simulink model "Sim_Modell_hydraulisches_System_2015a"  (R2015a)
settings: Solver=ode15s  StartTime=0.0  StopTime=10  RelTol=1e-6  AbsTol=1e-5
InitFcn:
  | Parameter_hydraulisches_System
undefined symbols (not defined in the file or in its folder): parImp, parRegA, parRegoA, parSys
libraries: simulink x4, cstblocks x2
settings Model: Creator=wke  LastModifiedBy=danielhauer
settings DataIOCC: SignalLoggingSaveFormat=ModelDataLogs
settings OptimizationCC: ExpressionDepthLimit=2147483647  InitFltsAndDblsToZero=on
settings DebuggingCC: UnderspecifiedInitializationDetection=Classic  MergeDetectMultiDrivingBlocksExec=none  SolverPrmCheckMsg=warning  FcnCallInpInsideContextMsg=UseLocalSettings  StateNameClashWarn=warning
settings SFSimCC: SimParseCustomCode=off
settings GRTTargetCC: CombineOutputUpdateFcns=off  GRTInterface=on

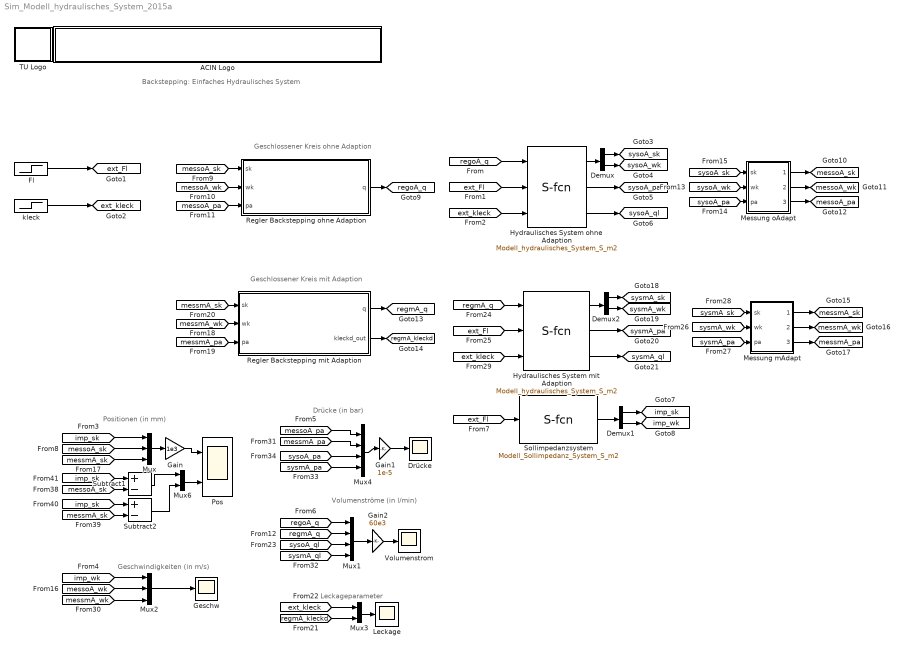
== system Sim_Modell_hydraulisches_System_2015a ==
  note: Positionen (in mm)
  note: Geschwindigkeiten (in m/s)
  note: Drücke (in bar)
  note: Leckageparameter
  note: Volumenströme (in l/min)
  note: Geschlossener Kreis ohne Adaption
  note: Geschlossener Kreis mit Adaption
  note: Backstepping: Einfaches Hydraulisches System
  ACIN Logo : Subsystem
      mask init:
      | s = get_param(gcb,'UserData');
      mask Display:
      | image(s.logo,[0 0 439 45]);
      | %axis image
  Demux : Demux  Outputs=2
  Demux1 : Demux  Outputs=2
  Demux2 : Demux  Outputs=2
  Drücke : Scope
      settings: TimeRange=auto  MaxDataPoints=5000  SaveToWorkspace=off  SaveName=ScopeData2  YMin=-10  YMax=10  SampleTime=-1
  Fl : Step  Time=3  After=1e4  SampleTime=0
  Gain : Gain  Gain=1e3
  Gain1 : Gain  Gain=1e-5
  Gain2 : Gain  Gain=60e3
  Geschw : Scope
      settings: TimeRange=auto  MaxDataPoints=5000  SaveToWorkspace=off  YMin=-10  YMax=10  SampleTime=-1
  "Hydraulisches System mit Adaption " : M-S-Function  FunctionName=Modell_hydraulisches_System_S_m2  Parameters=Aa_par,Ab_par,V0a_par,pb_par,beta_par,dk_par,m_par,sk0_par,wk0_par,pa0_par  mask{Aa_par=parSys.Aa, Ab_par=parSys.Ab, V0a_par=parSys.V0a, pb_par=parSys.pb, beta_par=parSys.beta, dk_par=parSys.dk, m_par=parSys.m, sk0_par=parSys.sk0, wk0_par=parSys.wk0, pa0_par=parSys.pa0}
      mask prompts: Aa_par "Druckwirksame Fläche Kolbenseite"; Ab_par "Druckwirksame Fläche Stangenseite"; V0a_par "eff. Volumen Kolbenseite für sk=0"; pb_par "Vorspanndruck Stangeseite"; beta_par "Kompressionsmodul"; dk_par "visk. Reibung des Kolbens"; m_par "eff. Masse des Kolbens mit Last"; sk0_par "Anfangsbedingung sk"; wk0_par "Anfangsbedingung wk"; pa0_par "Anfangsbedingung pa"
      mask Display:
      | port_label('input',1,'q');
      | port_label('input',2,'Fl');
      | port_label('input',3,'kl');
      | port_label('output',1,'sk, wk');
      | port_label('output',2,'pa');
      | port_label('output',3,'ql');
  Hydraulisches System ohne Adaption : M-S-Function  FunctionName=Modell_hydraulisches_System_S_m2  Parameters=Aa_par,Ab_par,V0a_par,pb_par,beta_par,dk_par,m_par,sk0_par,wk0_par,pa0_par  mask{Aa_par=parSys.Aa, Ab_par=parSys.Ab, V0a_par=parSys.V0a, pb_par=parSys.pb, beta_par=parSys.beta, dk_par=parSys.dk, m_par=parSys.m, sk0_par=parSys.sk0, wk0_par=parSys.wk0, pa0_par=parSys.pa0}
      mask prompts: Aa_par "Druckwirksame Fläche Kolbenseite"; Ab_par "Druckwirksame Fläche Stangenseite"; V0a_par "eff. Volumen Kolbenseite für sk=0"; pb_par "Vorspanndruck Stangeseite"; beta_par "Kompressionsmodul"; dk_par "visk. Reibung des Kolbens"; m_par "eff. Masse des Kolbens mit Last"; sk0_par "Anfangsbedingung sk"; wk0_par "Anfangsbedingung wk"; pa0_par "Anfangsbedingung pa"
      mask Display:
      | port_label('input',1,'q');
      | port_label('input',2,'Fl');
      | port_label('input',3,'kl');
      | port_label('output',1,'sk, wk');
      | port_label('output',2,'pa');
      | port_label('output',3,'ql');
  Leckage : Scope
      settings: TimeRange=auto  MaxDataPoints=5000  SaveToWorkspace=off  SaveName=ScopeData8  YMin=1.6e-012  YMax=3.9e-012  SampleTime=-1
  Messung mAdapt : Subsystem  mask{rauschenein_par=off, rauschampl_sk=5e-4, rauschampl_pa=5e4}
      mask prompts: rauschenein_par "Rauschen ein"; rauschampl_sk "Rauschamplitude Position sk"; rauschampl_pa "Rauschamplitude Druck pa"
  Messung oAdapt : Subsystem  mask{rauschenein_par=off, rauschampl_sk=5e-4, rauschampl_pa=5e4}
      mask prompts: rauschenein_par "Rauschen ein"; rauschampl_sk "Rauschamplitude Position sk"; rauschampl_pa "Rauschamplitude Druck pa"
  Mux : Mux  Inputs=3
  Mux1 : Mux
  Mux2 : Mux  Inputs=3
  Mux3 : Mux  Inputs=2
  Mux4 : Mux
  Mux6 : Mux  Inputs=2
  Pos : Scope  NumInputPorts=2
      settings: TimeRange=auto  MaxDataPoints=5000  SaveToWorkspace=off  SaveName=ScopeData  YMin=-0.4~-0.0004  YMax=0.4~0.0004  SampleTime=-1
  Regler Backstepping mit Adaption : MATLAB Function  TreatAsAtomicUnit=on
      settings: PermitHierarchicalResolution=ParametersOnly
  Regler Backstepping ohne Adaption : MATLAB Function  TreatAsAtomicUnit=on
      settings: PermitHierarchicalResolution=ParametersOnly
  Sollimpedanzsystem : M-S-Function  FunctionName=Modell_Sollimpedanz_System_S_m2  Parameters=m_par,c1I_par,c3I_par,c0I_par,skImax_par,numFeder_par,d1I_par,skI0_par,wkI0_par  mask{m_par=parSys.m, c1I_par=parImp.c1I, c3I_par=parImp.c3I, c0I_par=parImp.c0I, skImax_par=parImp.skImax, numFeder_par=parImp.numFeder, d1I_par=parImp.d1I, skI0_par=parSys.sk0, wkI0_par=parSys.wk0}
      mask prompts: m_par "eff. Masse des Kolbens mit Last"; c1I_par "lineare Steifigkeit"; c3I_par "kubische Steifigkeit"; c0I_par "Steifigkeit tan Feder"; skImax_par "max Auslenkung tan Feder"; numFeder_par "Auswahl der Feder"; d1I_par "visk. Dämpfung"; skI0_par "Anfangsbedingung skI"; wkI0_par "Anfangsbedingung wkI"
      mask Display:
      | port_label('input',1,'Fl');
      | port_label('output',1,'skI, wkI');
  Subtract1 : Sum  Inputs=+-
  Subtract2 : Sum  Inputs=+-
  TU Logo : Subsystem
      mask init:
      | s = get_param(gcb,'UserData');
      mask Display: image(s.logo,[0 0 45 45]);
  Volumenstrom : Scope
      settings: TimeRange=auto  MaxDataPoints=5000  SaveToWorkspace=off  SaveName=ScopeData3  YMin=-150  YMax=100  SampleTime=-1
  kleck : Step  Before=parSys.klecknom*1  After=parSys.klecknom  SampleTime=0
  tag scope: ext_Fl=global, ext_kleck=global, imp_sk=global, imp_wk=global, messmA_pa=global, messmA_sk=global, messmA_wk=global, messoA_pa=global, messoA_sk=global, messoA_wk=global, regmA_kleckd=global, regmA_q=global, regoA_q=global, sysmA_pa=global, sysmA_ql=global, sysmA_sk=global, sysmA_wk=global, sysoA_pa=global, sysoA_ql=global, sysoA_sk=global, sysoA_wk=global
  wires:
  [regoA_q] -> Hydraulisches System ohne Adaption/1
  Fl/1 -> [ext_Fl]
  kleck/1 -> [ext_kleck]
  [ext_Fl] -> Hydraulisches System ohne Adaption/2
  [ext_kleck] -> Hydraulisches System ohne Adaption/3
  Hydraulisches System ohne Adaption/1 -> Demux/1
  Demux/1 -> [sysoA_sk]
  Demux/2 -> [sysoA_wk]
  Hydraulisches System ohne Adaption/2 -> [sysoA_pa]
  Gain/1 -> Pos/1
  Gain1/1 -> Drücke/1
  Gain2/1 -> Volumenstrom/1
  Demux1/1 -> [imp_sk]
  Demux1/2 -> [imp_wk]
  Sollimpedanzsystem/1 -> Demux1/1
  [ext_Fl] -> Sollimpedanzsystem/1
  Mux/1 -> Gain/1
  [imp_sk] -> Mux/1
  [messoA_sk] -> Mux/2
  Regler Backstepping ohne Adaption/1(q) -> [regoA_q]
  [messoA_wk] -> Regler Backstepping ohne Adaption/2(wk)
  [messoA_sk] -> Regler Backstepping ohne Adaption/1(sk)
  [messoA_pa] -> Regler Backstepping ohne Adaption/3(pa)
  [regoA_q] -> Mux1/1
  Mux1/1 -> Gain2/1
  [regmA_q] -> Mux1/2
  [sysoA_sk] -> Messung oAdapt/1(sk)
  [sysoA_wk] -> Messung oAdapt/2(wk)
  [sysoA_pa] -> Messung oAdapt/3(pa)
  Messung oAdapt/3(pamess) -> [messoA_pa]
  Messung oAdapt/2(wkmess) -> [messoA_wk]
  Messung oAdapt/1(skmess) -> [messoA_sk]
  [imp_wk] -> Mux2/1
  Mux2/1 -> Geschw/1
  [messoA_wk] -> Mux2/2
  [messmA_sk] -> Mux/3
  [messmA_wk] -> Regler Backstepping mit Adaption/2(wk)
  [messmA_sk] -> Regler Backstepping mit Adaption/1(sk)
  [messmA_pa] -> Regler Backstepping mit Adaption/3(pa)
  Regler Backstepping mit Adaption/2(kleckd_out) -> [regmA_kleckd]
  Regler Backstepping mit Adaption/1(q) -> [regmA_q]
  [ext_kleck] -> Mux3/1
  Mux3/1 -> Leckage/1
  [regmA_kleckd] -> Mux3/2
  [sysoA_ql] -> Mux1/3
  [regmA_q] -> "Hydraulisches System mit Adaption "/1
  [ext_Fl] -> "Hydraulisches System mit Adaption "/2
  [ext_kleck] -> "Hydraulisches System mit Adaption "/3
  "Hydraulisches System mit Adaption "/1 -> Demux2/1
  Demux2/1 -> [sysmA_sk]
  Demux2/2 -> [sysmA_wk]
  "Hydraulisches System mit Adaption "/3 -> [sysmA_ql]
  [sysmA_sk] -> Messung mAdapt/1(sk)
  [sysmA_wk] -> Messung mAdapt/2(wk)
  [sysmA_pa] -> Messung mAdapt/3(pa)
  Messung mAdapt/3(pamess) -> [messmA_pa]
  Messung mAdapt/2(wkmess) -> [messmA_wk]
  Messung mAdapt/1(skmess) -> [messmA_sk]
  [messmA_wk] -> Mux2/3
  [messoA_pa] -> Mux4/1
  [messmA_pa] -> Mux4/2
  Mux4/1 -> Gain1/1
  [sysmA_ql] -> Mux1/4
  [sysoA_pa] -> Mux4/3
  [sysmA_pa] -> Mux4/4
  Hydraulisches System ohne Adaption/3 -> [sysoA_ql]
  "Hydraulisches System mit Adaption "/2 -> [sysmA_pa]
  [imp_sk] -> Subtract1/1
  [messoA_sk] -> Subtract1/2
  [imp_sk] -> Subtract2/1
  [messmA_sk] -> Subtract2/2
  Subtract2/1 -> Mux6/2
  Subtract1/1 -> Mux6/1
  Mux6/1 -> Pos/2

== system Sim_Modell_hydraulisches_System_2015a/ACIN Logo ==

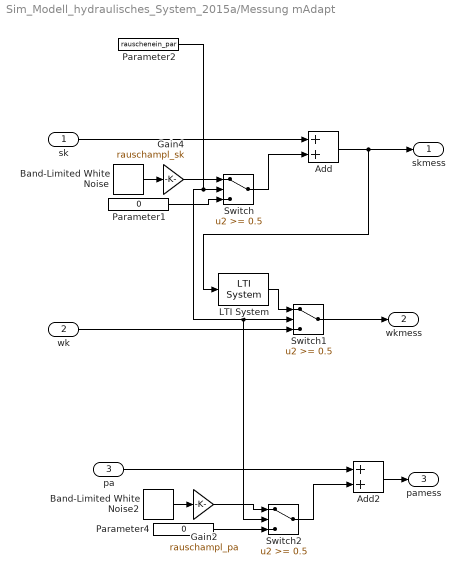
== system Sim_Modell_hydraulisches_System_2015a/Messung mAdapt ==
  sk : Inport
  wk : Inport  Port=2
  pa : Inport  Port=3
  Add : Sum
  Add2 : Sum
  Band-Limited White Noise : simulink/Sources/Band-Limited White Noise  Cov=[0.0001]  Ts=0.001  seed=[23341]
  Band-Limited White Noise2 : simulink/Sources/Band-Limited White Noise  Cov=[0.0001]  Ts=0.001  seed=[23341]
  Gain2 : Gain  Gain=rauschampl_pa
  Gain4 : Gain  Gain=rauschampl_sk
  LTI System : cstblocks/LTI System  sys=parMess.Gdiffsk  IC=[]
  Parameter1 : Constant  Value=0  VectorParams1D=off
  Parameter2 : Constant  Value=rauschenein_par  VectorParams1D=off
  Parameter4 : Constant  Value=0  VectorParams1D=off
  Switch : Switch  Threshold=0.5
  Switch1 : Switch  Threshold=0.5
  Switch2 : Switch  Threshold=0.5
  skmess : Outport
  wkmess : Outport  Port=2
  pamess : Outport  Port=3
  wires:
  Parameter1/1 -> Switch/3
  Gain4/1 -> Switch/1
  wk/1 -> Switch1/3
  LTI System/1 -> Switch1/1
  Gain2/1 -> Switch2/1
  Parameter4/1 -> Switch2/3
  Switch1/1 -> wkmess/1
  Add2/1 -> pamess/1
  pa/1 -> Add2/1
  Switch2/1 -> Add2/2
  Band-Limited White Noise2/1 -> Gain2/1
  Add/1 -> LTI System/1, skmess/1
  sk/1 -> Add/1
  Parameter2/1 -> Switch2/2, Switch1/2, Switch/2
  Switch/1 -> Add/2
  Band-Limited White Noise/1 -> Gain4/1

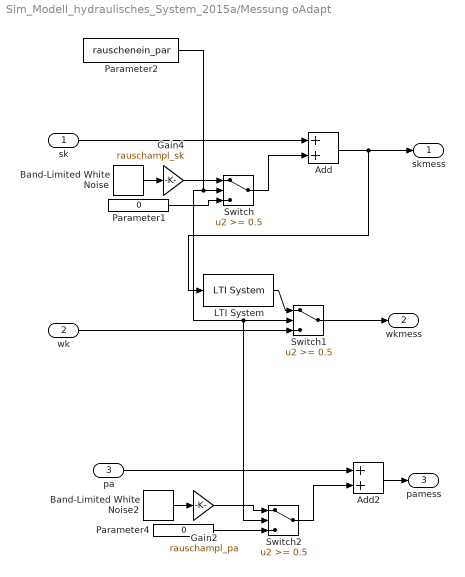
== system Sim_Modell_hydraulisches_System_2015a/Messung oAdapt ==
  sk : Inport
  wk : Inport  Port=2
  pa : Inport  Port=3
  Add : Sum
  Add2 : Sum
  Band-Limited White Noise : simulink/Sources/Band-Limited White Noise  Cov=[0.0001]  Ts=0.001  seed=[23341]
  Band-Limited White Noise2 : simulink/Sources/Band-Limited White Noise  Cov=[0.0001]  Ts=0.001  seed=[23341]
  Gain2 : Gain  Gain=rauschampl_pa
  Gain4 : Gain  Gain=rauschampl_sk
  LTI System : cstblocks/LTI System  sys=parMess.Gdiffsk  IC=[]
  Parameter1 : Constant  Value=0  VectorParams1D=off
  Parameter2 : Constant  Value=rauschenein_par  VectorParams1D=off
  Parameter4 : Constant  Value=0  VectorParams1D=off
  Switch : Switch  Threshold=0.5
  Switch1 : Switch  Threshold=0.5
  Switch2 : Switch  Threshold=0.5
  skmess : Outport
  wkmess : Outport  Port=2
  pamess : Outport  Port=3
  wires:
  Band-Limited White Noise/1 -> Gain4/1
  Switch/1 -> Add/2
  Parameter2/1 -> Switch/2, Switch1/2, Switch2/2
  sk/1 -> Add/1
  Add/1 -> skmess/1, LTI System/1
  Band-Limited White Noise2/1 -> Gain2/1
  Switch2/1 -> Add2/2
  pa/1 -> Add2/1
  Add2/1 -> pamess/1
  Switch1/1 -> wkmess/1
  Parameter4/1 -> Switch2/3
  Gain2/1 -> Switch2/1
  LTI System/1 -> Switch1/1
  wk/1 -> Switch1/3
  Gain4/1 -> Switch/1
  Parameter1/1 -> Switch/3

== system Sim_Modell_hydraulisches_System_2015a/TU Logo ==

== matlab function Sim_Modell_hydraulisches_System_2015a/Regler Backstepping mit Adaption ==
  settings: updateMethod=DISCRETE  sampleTime=parRegA.Ts
  data sk settings: updateMethod=SF_CONTINUOUS_TIME_DATA
  data wk settings: updateMethod=SF_CONTINUOUS_TIME_DATA
  data pa settings: updateMethod=SF_CONTINUOUS_TIME_DATA
  data parSys settings: updateMethod=SF_CONTINUOUS_TIME_DATA
  data q settings: updateMethod=SF_CONTINUOUS_TIME_DATA
  data: sk input; wk input; pa input; parSys parameter; q output; kleckd_out output; parImp parameter; parRegA parameter
function [q,kleckd_out]  = Backstepping_mit_Adapt(sk,wk,pa,parSys,parImp, parRegA)
% Funktion zur Implementierung eines Backsteppingreglers mit
% Adaption für einfaches hydraulisches System


% Initialisierung des diskreten Integrator Zustandes
persistent kleckd
if isempty(kleckd) kleckd = parSys.klecknom; end

% Zuweisung der Parameter

m = parSys.m;
dk = parSys.dk;
beta = parSys.beta;
Aa = parSys.Aa;
Ab = parSys.Ab;
V0a = parSys.V0a;
pb = parSys.pb;


c1I = parImp.c1I;
c3I = parImp.c3I;
c0I= parImp.c0I;
skImax = parImp.skImax;
d1I = parImp.d1I;
numFeder = parImp.numFeder;

k0=parRegA.k0;
k1= parRegA.k1;
gamma = parRegA.gamma;

%Berechnung von Fp aus pa und pb
Fp=pa*Aa-pb*Ab;

%Berechnung der Einträge des Systems
f1=[wk;-dk/m*wk];
g1=[0;1/m];
f2dach=[beta*Aa/(V0a+Aa*sk)*(-Aa*wk-kleckd/Aa*(Fp-pb*(Aa-Ab)))];
g2=[beta*Aa/(V0a+Aa*sk)];
x1=[sk;wk];
x2=[Fp];

%Bestimmung der Federkraft und der Ableitung der Federkraft
if numFeder<1.5
    FcI=c1I*sk;      %lineare Feder
    dFcIdsk=c1I;
elseif numFeder<2.5
    FcI=c1I*sk+c3I*sk^3;
    dFcIdsk=c1I+3*c3I*sk^2;
else
    FcI=c0I*2*skImax/pi*tan(pi*sk/2/skImax);
    dFcIdsk=c0I*(1+(tan(pi*sk/2/skImax))^2);
end;

%Berechnung von alpha1 und dalpha1/dx1
alpha1=-FcI-(d1I-dk)*wk;
dalpha1dx1=[-dFcIdsk,-(d1I-dk)];

%Berechnung von dV1dx1
dV1dx1=[FcI,m*wk];

%Berechnung des Stellgesetzes
q=1/g2*(-f2dach+dalpha1dx1*(f1+g1*x2)-dV1dx1*g1/gamma-k1*(x2-alpha1));

%Berechnung des Parameterschätzers
kleckd_out = kleckd; % Ausgabe des aktuellen Zustandes

chi=beta/(V0a+Aa*sk)*(Fp-pb*(Aa-Ab));
dkleckddt=-k0*(x2-alpha1)*chi;
% Zeitdiskreter Intergratorschritt nach Euler-Vorwärts
kleckd = kleckd + parRegA.Ts*dkleckddt;

== matlab function Sim_Modell_hydraulisches_System_2015a/Regler Backstepping ohne Adaption ==
  data sk settings: updateMethod=SF_CONTINUOUS_TIME_DATA
  data wk settings: updateMethod=SF_CONTINUOUS_TIME_DATA
  data pa settings: updateMethod=SF_CONTINUOUS_TIME_DATA
  data parSys settings: updateMethod=SF_CONTINUOUS_TIME_DATA
  data q settings: updateMethod=SF_CONTINUOUS_TIME_DATA
  data: sk input; wk input; pa input; parSys parameter; q output; parRegoA parameter; parImp parameter
function q  = Backstepping_ohne_Adapt(sk,wk,pa,parSys, parRegoA, parImp)
% Funktion zur Implementierung eines Backsteppingreglers ohne
% Adaption für einfaches hydraulisches System

% Zuweisung der Parameter

m = parSys.m;
dk = parSys.dk;
beta = parSys.beta;
Aa = parSys.Aa;
Ab = parSys.Ab;
V0a = parSys.V0a;
pb = parSys.pb;
klecknom = parSys.klecknom;

c1I = parImp.c1I;
c3I = parImp.c3I;
c0I= parImp.c0I;
skImax = parImp.skImax;
d1I = parImp.d1I;
numFeder = parImp.numFeder;

k1= parRegoA.k1;
gamma = parRegoA.gamma;

%Berechnung von Fp aus pa und pb
Fp=pa*Aa-pb*Ab;

%Berechnung der Einträge des Systems
f1=[wk;-dk/m*wk];
g1=[0;1/m];
f2=[beta*Aa/(V0a+Aa*sk)*(-Aa*wk-klecknom/Aa*(Fp-pb*(Aa-Ab)))];
g2=[beta*Aa/(V0a+Aa*sk)];
x1=[sk;wk];
x2=[Fp];

%Bestimmung der Federkraft und der Ableitung der Federkraft
if numFeder<1.5
    FcI=c1I*sk;      %lineare Feder
    dFcIdsk=c1I;
elseif numFeder<2.5
    FcI=c1I*sk+c3I*sk^3;
    dFcIdsk=c1I+3*c3I*sk^2;
else
    FcI=c0I*2*skImax/pi*tan(pi*sk/2/skImax);
    dFcIdsk=c0I*(1+(tan(pi*sk/2/skImax))^2);
end;

%Berechnung von alpha1 und dalpha1/dx1
alpha1=-FcI-(d1I-dk)*wk;
dalpha1dx1=[-dFcIdsk,-(d1I-dk)];

%Berechnung von dV1dx1
 dV1dx1=[FcI,m*wk];


%Berechnung des Stellgesetzes
q=1/g2*(-f2+dalpha1dx1*(f1+g1*x2)-dV1dx1*g1/gamma-k1*(x2-alpha1));
